simulink library "Over_Current_Protection_Relay"  (R2024a)
settings: Solver=VariableStepAuto  StartTime=0.0  StopTime=10.0  RelTol=1e-3
libraries: spsCurrentMeasurementLib x3, simulink_extras x3, spsThreePhaseBreakerLib x1
settings Model: Creator=gshma  LastModifiedBy=gshma

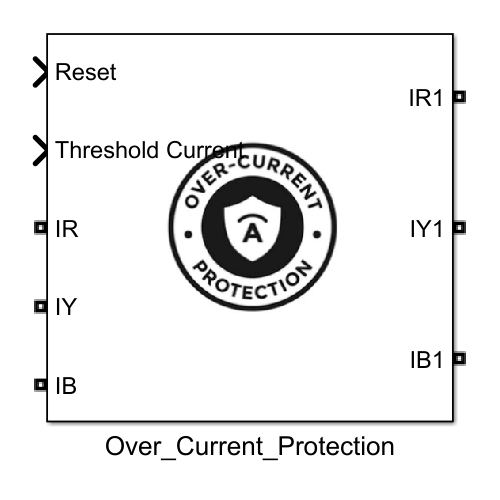
[thumbnail: Simulink's stored preview of the top-level diagram]
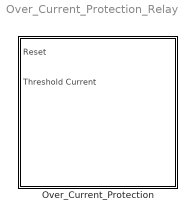
== system Over_Current_Protection_Relay ==
  Over_Current_Protection : Subsystem
      mask Display: image('ovc.png', [0,0,0,0,50,50]);

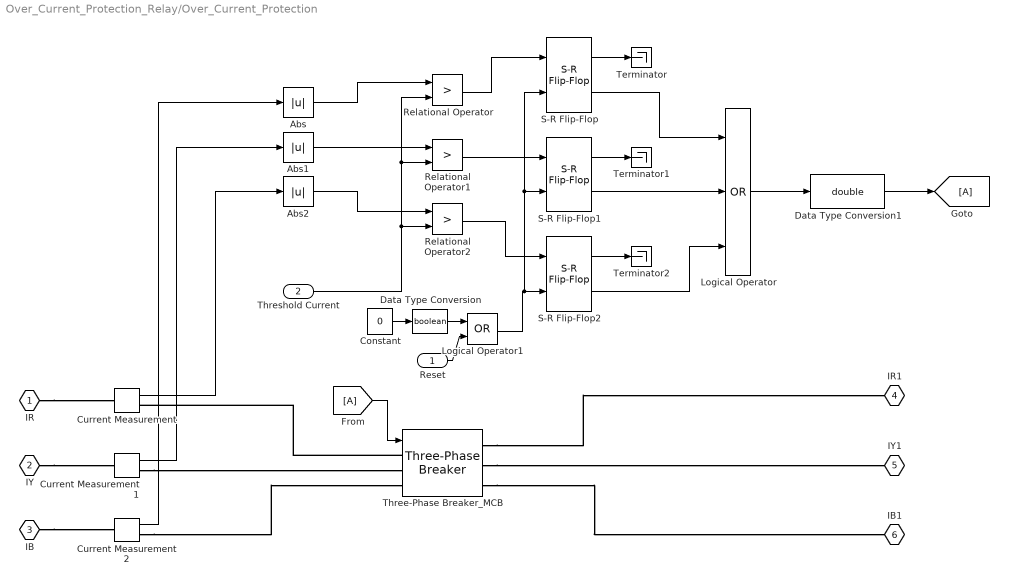
== system Over_Current_Protection_Relay/Over_Current_Protection ==
  Reset : Inport
  Threshold Current : Inport  Port=2
  Abs : Abs  SaturateOnIntegerOverflow=off
  Abs1 : Abs  SaturateOnIntegerOverflow=off
  Abs2 : Abs  SaturateOnIntegerOverflow=off
  Constant : Constant  Value=0  SampleTime=0.001
  Current Measurement : spsCurrentMeasurementLib/Current Measurement  PhasorSimulation=off  OutputType=Complex  PSBequivalent=0
  Current Measurement1 : spsCurrentMeasurementLib/Current Measurement  PhasorSimulation=off  OutputType=Complex  PSBequivalent=0
  Current Measurement2 : spsCurrentMeasurementLib/Current Measurement  PhasorSimulation=off  OutputType=Complex  PSBequivalent=0
  Data Type Conversion : DataTypeConversion  OutDataTypeStr=boolean  SaturateOnIntegerOverflow=off  RndMeth=Floor
  Data Type Conversion1 : DataTypeConversion  OutDataTypeStr=double  SaturateOnIntegerOverflow=off  RndMeth=Floor
  From : From
  Goto : Goto
  Logical Operator : Logic  Operator=OR  Inputs=3  AllPortsSameDT=off  OutDataTypeStr=boolean
  Logical Operator1 : Logic  Operator=OR  AllPortsSameDT=off  OutDataTypeStr=boolean
  Relational Operator : RelationalOperator  Operator=>  OutDataTypeStr=boolean  RndMeth=Simplest  InputSameDT=off
  Relational Operator1 : RelationalOperator  Operator=>  OutDataTypeStr=boolean  RndMeth=Simplest  InputSameDT=off
  Relational Operator2 : RelationalOperator  Operator=>  OutDataTypeStr=boolean  RndMeth=Simplest  InputSameDT=off
  S-R Flip-Flop : simulink_extras/Flip Flops/S-R Flip-Flop  initial_condition=0
  S-R Flip-Flop1 : simulink_extras/Flip Flops/S-R Flip-Flop  initial_condition=0
  S-R Flip-Flop2 : simulink_extras/Flip Flops/S-R Flip-Flop  initial_condition=0
  Terminator : Terminator
  Terminator1 : Terminator
  Terminator2 : Terminator
  Three-Phase Breaker_MCB : spsThreePhaseBreakerLib/Three-Phase Breaker  InitialState=closed  SwitchA=on  SwitchB=on  SwitchC=on  SwitchTimes="[1/60  5/60]"  External=on  BreakerResistance=0.01  SnubberResistance=1e6  SnubberCapacitance=inf  Measurements=None
  IR : PMIOPort  Tag=simrfV2util1/Connection Port  Side=Left
  IY : PMIOPort  Tag=simrfV2util1/Connection Port  Port=2  Side=Left
  IB : PMIOPort  Tag=simrfV2util1/Connection Port  Port=3  Side=Left
  IR1 : PMIOPort  Tag=simrfV2util1/Connection Port  Port=4  Side=Right
  IY1 : PMIOPort  Tag=simrfV2util1/Connection Port  Port=5  Side=Right
  IB1 : PMIOPort  Tag=simrfV2util1/Connection Port  Port=6  Side=Right
  wires:
  Current Measurement/1 -> Abs2/1
  Current Measurement1/1 -> Abs1/1
  Current Measurement2/1 -> Abs/1
  Abs2/1 -> Relational Operator2/1
  Abs1/1 -> Relational Operator1/1
  Abs/1 -> Relational Operator/1
  Threshold Current/1 -> Relational Operator2/2, Relational Operator1/2, Relational Operator/2
  Relational Operator/1 -> S-R Flip-Flop/1
  Relational Operator1/1 -> S-R Flip-Flop1/1
  Relational Operator2/1 -> S-R Flip-Flop2/1
  Constant/1 -> Data Type Conversion/1
  S-R Flip-Flop/2 -> Logical Operator/1
  S-R Flip-Flop1/2 -> Logical Operator/2
  S-R Flip-Flop2/2 -> Logical Operator/3
  S-R Flip-Flop2/1 -> Terminator2/1
  S-R Flip-Flop1/1 -> Terminator1/1
  S-R Flip-Flop/1 -> Terminator/1
  From/1 -> Three-Phase Breaker_MCB/1
  Logical Operator/1 -> Data Type Conversion1/1
  Data Type Conversion1/1 -> Goto/1
  Reset/1 -> Logical Operator1/2
  Logical Operator1/1 -> S-R Flip-Flop/2, S-R Flip-Flop1/2, S-R Flip-Flop2/2
  Data Type Conversion/1 -> Logical Operator1/1
  connections:
  IR/RConn1 -- Current Measurement/LConn1
  IY/RConn1 -- Current Measurement1/LConn1
  IB/RConn1 -- Current Measurement2/LConn1
  Three-Phase Breaker_MCB/LConn1 -- Current Measurement/RConn1
  Current Measurement1/RConn1 -- Three-Phase Breaker_MCB/LConn2
  Current Measurement2/RConn1 -- Three-Phase Breaker_MCB/LConn3
  Three-Phase Breaker_MCB/RConn1 -- IR1/RConn1
  Three-Phase Breaker_MCB/RConn2 -- IY1/RConn1
  Three-Phase Breaker_MCB/RConn3 -- IB1/RConn1
